simulink model "Simulador_Dinamica"  (R2024b)
settings: Solver=VariableStepAuto  StartTime=0.0  StopTime=4  RelTol=1e-3
settings Model: Creator=aleja  LastModifiedBy=aleja
settings DataIOCC: ReturnWorkspaceOutputs=off

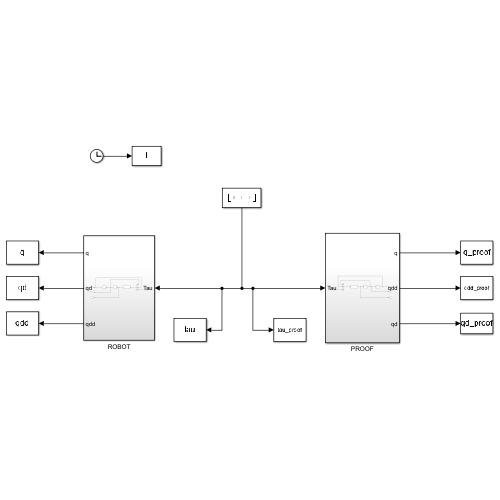
[thumbnail: Simulink's stored preview of the top-level diagram]
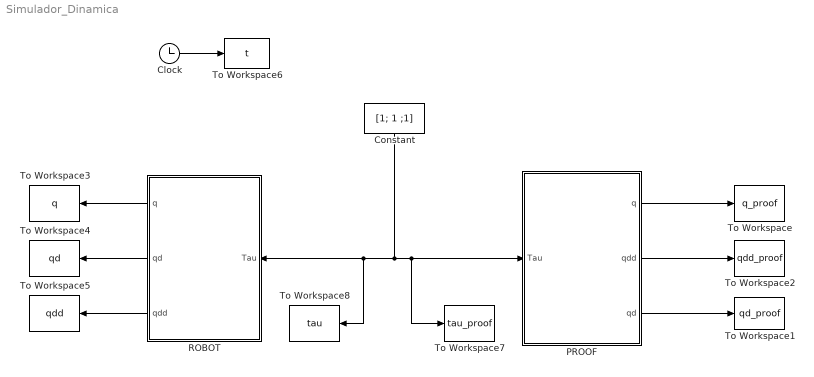
== system Simulador_Dinamica ==
  Clock : Clock
      settings: Decimation=4
  Constant : Constant  Value=[1; 1 ;1]
  PROOF : Subsystem
  ROBOT : Subsystem
  To Workspace : ToWorkspace  VariableName=q_proof  SampleTime=-1
  To Workspace1 : ToWorkspace  VariableName=qd_proof  SampleTime=-1
  To Workspace2 : ToWorkspace  VariableName=qdd_proof  SampleTime=-1
  To Workspace3 : ToWorkspace  VariableName=q  SampleTime=-1
  To Workspace4 : ToWorkspace  VariableName=qd  SampleTime=-1
  To Workspace5 : ToWorkspace  VariableName=qdd  SampleTime=-1
  To Workspace6 : ToWorkspace  VariableName=t  SaveFormat=Timeseries  SampleTime=-1
  To Workspace7 : ToWorkspace  VariableName=tau_proof  SaveFormat=Timeseries  SampleTime=-1
  To Workspace8 : ToWorkspace  VariableName=tau  SaveFormat=Timeseries  SampleTime=-1
  wires:
  Constant/1 -> To Workspace8/1, ROBOT/1(Tau), To Workspace7/1, PROOF/1(Tau)
  PROOF/3(qd) -> To Workspace1/1
  ROBOT/1(q) -> To Workspace3/1
  ROBOT/2(qd) -> To Workspace4/1
  ROBOT/3(qdd) -> To Workspace5/1
  PROOF/2(qdd) -> To Workspace2/1
  PROOF/1(q) -> To Workspace/1
  Clock/1 -> To Workspace6/1

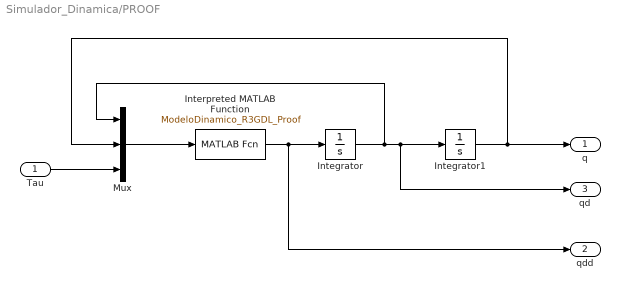
== system Simulador_Dinamica/PROOF ==
  Tau : Inport
  Integrator : Integrator
  Integrator1 : Integrator
  Interpreted MATLAB Function : MATLABFcn  MATLABFcn=ModeloDinamico_R3GDL_Proof  OutputDimensions=3
  Mux : Mux  Inputs=3
  q : Outport
  qdd : Outport  Port=2
  qd : Outport  Port=3
  wires:
  Mux/1 -> Interpreted MATLAB Function/1
  Tau/1 -> Mux/3
  Interpreted MATLAB Function/1 -> qdd/1, Integrator/1
  Integrator/1 -> Mux/1, qd/1, Integrator1/1
  Integrator1/1 -> Mux/2, q/1

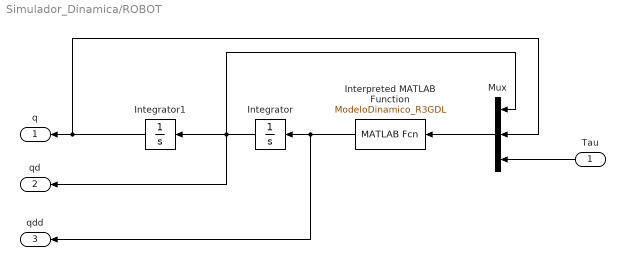
== system Simulador_Dinamica/ROBOT ==
  Tau : Inport
  Integrator : Integrator
  Integrator1 : Integrator
  Interpreted MATLAB Function : MATLABFcn  MATLABFcn=ModeloDinamico_R3GDL  OutputDimensions=3
  Mux : Mux  Inputs=3
  q : Outport
  qd : Outport  Port=2
  qdd : Outport  Port=3
  wires:
  Tau/1 -> Mux/3
  Integrator1/1 -> Mux/2, q/1
  Interpreted MATLAB Function/1 -> qdd/1, Integrator/1
  Integrator/1 -> Mux/1, qd/1, Integrator1/1
  Mux/1 -> Interpreted MATLAB Function/1
